simulink model "q3_p1"  (R2022a)
settings: Solver=FixedStepDiscrete  StartTime=0.0  StopTime=10.0  RelTol=1e-3  EnableMultiTasking=on
settings Model: ExtModeTrigDuration=2  Creator=Amin  LastModifiedBy=Amin
settings OptimizationCC: EnhancedBackFolding=on  PassReuseOutputArgsAs=Individual arguments  ZeroExternalMemoryAtStartup=off  ZeroInternalMemoryAtStartup=off  MaxStackSize=64  OptimizeBlockOrder=speed  DifferentSizesBufferReuse=on  OptimizationCustomize=off  EfficientTunableParamExpr=on
settings DebuggingCC: SignalRangeChecking=warning  ParameterTunabilityLossMsg=error
settings HardwareCC: ProdBitPerInt=16  ProdBitPerPointer=16  ProdBitPerSizeT=16  ProdBitPerPtrDiffT=16  ProdLargestAtomicFloat=None  ProdWordSize=8  ProdHWDeviceType=Atmel->AVR
settings SFSimCC: MATLABDynamicMemAlloc=off
settings RTWCC: SystemTargetFile=ert.tlc  HardwareBoard=Arduino Mega 2560  TemplateMakefile=ert_default_tmf  Toolchain=Arduino AVR  BuildConfiguration=Faster Runs
settings CodeAppCC: ForceParamTrailComments=on  IgnoreCustomStorageClasses=off  OperatorAnnotations=on  SimulinkDataObjDesc=on  SFDataObjDesc=on  InsertBlockDesc=on
settings ERTTargetCC: SupportContinuousTime=on  SupportVariableSizeSignals=on  ExtModeTransport=3  ExtModeStaticAlloc=on  ExtModeStaticAllocSize=2048  ExtModeMexFile=ext_xcp  ExtModeIntrfLevel=Level2 - Open

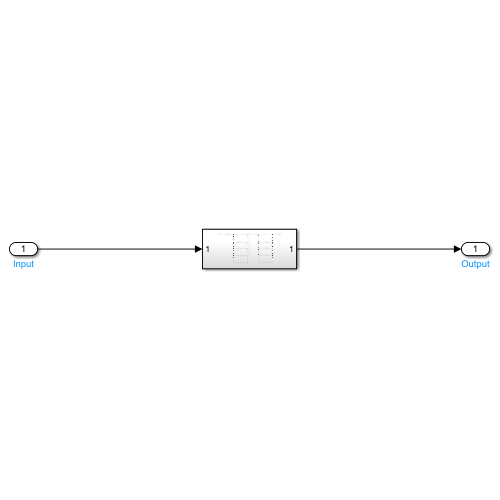
[thumbnail: Simulink's stored preview of the top-level diagram]
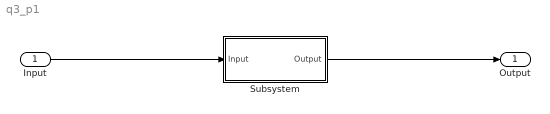
== system q3_p1 ==
  Input : Inport
  Subsystem : Subsystem
  Output : Outport
  wires:
  Input/1 -> Subsystem/1(Input)
  Subsystem/1(Output) -> Output/1

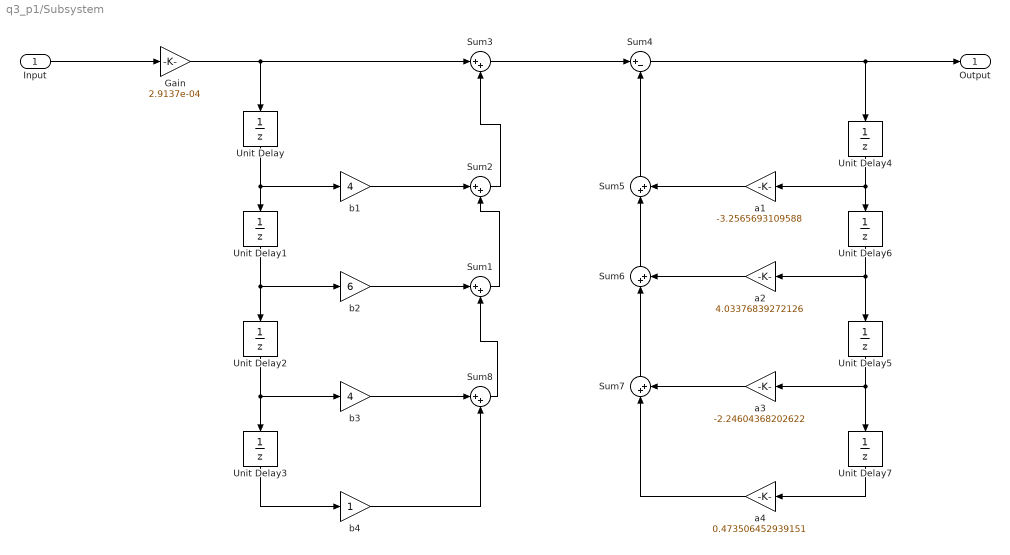
== system q3_p1/Subsystem ==
  Input : Inport
  Gain : Gain  Gain=2.9137e-04
  Sum{1..3,5..8} (7 alike) : Sum  Inputs=|++
  Sum4 : Sum  Inputs=|+-
  Unit Delay{,1..7} (8 alike) : UnitDelay  SampleTime=-1  HasFrameUpgradeWarning=on
  a1 : Gain  Gain=-3.2565693109588
  a2 : Gain  Gain=4.03376839272126
  a3 : Gain  Gain=-2.24604368202622
  a4 : Gain  Gain=0.473506452939151
  b1 : Gain  Gain=4
  b2 : Gain  Gain=6
  b3 : Gain  Gain=4
  b4 : Gain
  Output : Outport
  wires:
  b3/1 -> Sum8/1
  Unit Delay4/1 -> Unit Delay6/1, a1/1
  Input/1 -> Gain/1
  Sum4/1 -> Output/1, Unit Delay4/1
  Unit Delay/1 -> b1/1, Unit Delay1/1
  Unit Delay3/1 -> b4/1
  Sum1/1 -> Sum2/2
  a4/1 -> Sum7/1
  a1/1 -> Sum5/2
  a3/1 -> Sum7/2
  Sum8/1 -> Sum1/2
  Unit Delay6/1 -> a2/1, Unit Delay5/1
  b1/1 -> Sum2/1
  Sum5/1 -> Sum4/2
  Unit Delay5/1 -> a3/1, Unit Delay7/1
  a2/1 -> Sum6/2
  b4/1 -> Sum8/2
  b2/1 -> Sum1/1
  Unit Delay2/1 -> b3/1, Unit Delay3/1
  Sum7/1 -> Sum6/1
  Gain/1 -> Sum3/1, Unit Delay/1
  Sum2/1 -> Sum3/2
  Unit Delay1/1 -> b2/1, Unit Delay2/1
  Unit Delay7/1 -> a4/1
  Sum3/1 -> Sum4/1
  Sum6/1 -> Sum5/1
